simulink model "pfc"  (R2018b)
settings: Solver=VariableStepAuto  StartTime=0.0  StopTime=1  RelTol=1e-3
InitFcn:
  | % Time %
  | fpwm = 18e3
  | fs = fpwm
  | Ts = 1/fs
  | 
  | %pfc Current Loop - plant is only inductance%
  | Vin_ac = 264
  | Cin = 2.2e-6
  | Vin_peak = 1.414 * Vin_ac
  | Vin_dc = Vin_peak
  | Rshunt = 20e-3
  | L = 3e-3
  | R = 0.123
  | BW_Ipfc = 1400
  | Vmax = Vin_dc  % max applied Vplant %
  | Gain_Ipfc = (Vmax / 1)  % (Vplant / Ipfc_dutycycle) %
  | Kp_Ipfc = (2*pi*BW_Ipfc * L) / Gain_Ipfc
  | Ki_Ipfc = (2*pi*BW_Ipfc * R) / Gain_Ipfc
  | 
  | % pfc Voltage Loop %
  | Cdc = 1080e-6
  | Vc_init = 0.8*Vin_peak  % initial capacitor voltage %
  | Rload = 80
  | BW_Vpfc = 10
  | Gain_Vpfc = 1  % V_loop_PI_out to Iref_pfc %
  | Kp_Vpfc = (2*pi*BW_Vpfc * Cdc) / Gain_Vpfc
  | Ki_Vpfc = (2*pi*BW_Vpfc / Rload) / Gain_Vpfc
  | Gain_ffV = 0.25   % feed forward gain %
libraries: powerlib x17, dspstat3 x3, simulink x2, powerlib_meascontrol x1
settings Model: Creator=GURU SEKHAR  LastModifiedBy=GURU SEKHAR

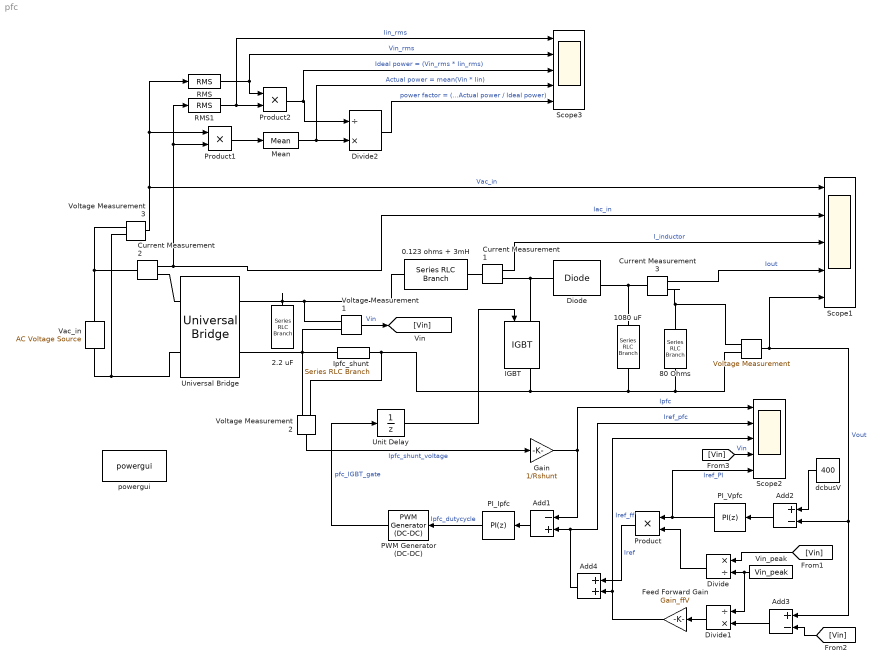
== system pfc ==
  "                       " : powerlib/Measurements/Voltage Measurement  PhasorSimulation=off  OutputType=Complex  PSBequivalent=0
  0.123 ohms + 3mH : powerlib/Elements/Series RLC Branch  LConnTagsString=__new0  RConnTagsString=__new0  BranchType=RL  Resistance=R  Inductance=L  SetiL0=off  InitialCurrent=0  Capacitance=1e-6  Setx0=off  InitialVoltage=0  Measurements=None
  1080 uF : powerlib/Elements/Series RLC Branch  LConnTagsString=__new0  RConnTagsString=__new0  BranchType=C  Resistance=1  Inductance=1e-3  SetiL0=off  InitialCurrent=0  Capacitance=Cdc  Setx0=on  InitialVoltage=Vc_init  Measurements=None
  2.2 uF : powerlib/Elements/Series RLC Branch  LConnTagsString=__new0  RConnTagsString=__new0  BranchType=C  Resistance=1  Inductance=1e-3  SetiL0=off  InitialCurrent=0  Capacitance=Cin  Setx0=off  InitialVoltage=Vc_init  Measurements=None
  "80 Ohms " : powerlib/Elements/Series RLC Branch  LConnTagsString=__new0  RConnTagsString=__new0  BranchType=R  Resistance=80  Inductance=1e-3  SetiL0=off  InitialCurrent=0  Capacitance=1e-6  Setx0=off  InitialVoltage=0  Measurements=None
  Add1 : Sum  Inputs=-+
  Add2 : Sum  Inputs=+-
  Add3 : Sum  Inputs=+-
  Add4 : Sum
  Current Measurement1 : powerlib/Measurements/Current Measurement  PhasorSimulation=off  OutputType=Complex  PSBequivalent=0
  Current Measurement2 : powerlib/Measurements/Current Measurement  PhasorSimulation=off  OutputType=Complex  PSBequivalent=0
  Current Measurement3 : powerlib/Measurements/Current Measurement  PhasorSimulation=off  OutputType=Complex  PSBequivalent=0
  Diode : powerlib/Power Electronics/Diode  Ron=0.001  Lon=0  Vf=0.8  IC=0  UseSnubber=off  Rs=500  Cs=250e-9  Measurements=on
  Divide : Product  Inputs=*/
  Divide1 : Product  Inputs=/*
  Divide2 : Product  Inputs=/*
  Feed Forward Gain : Gain  Gain=Gain_ffV
  Gain : Gain  Gain=1/Rshunt
  IGBT : powerlib/Power Electronics/IGBT  Ron=0.001  Lon=0  Vf=1  Tf=1e-6  Tt=2e-6  IC=0  Rs=1e5  Cs=inf  Measurements=on
  Ipfc_shunt : powerlib/Elements/Series RLC Branch  LConnTagsString=__new0  RConnTagsString=__new0  BranchType=R  Resistance=Rshunt  Inductance=1e-3  SetiL0=off  InitialCurrent=0  Capacitance=1e-6  Setx0=off  InitialVoltage=0  Measurements=None
  Mean : dspstat3/Mean  run=on  reset_popup=None  directionMode=Each column  dimension=1  roiEnable=off  roiType=Rectangles  roiPortion=Entire ROI  roiOutput=Individual statistics for each ROI  roiFlag=off  roundingMode=Floor  overflowMode=off  outputDataTypeStr=Inherit: Same as accumulator  outputMin=[]  outputMax=[]  outputLastDataTypeStr=Inherit: Same as accumulator
  PI_Ipfc : simulink/Continuous/PID Controller  Controller=PI  Form=Parallel  TimeDomain=Discrete-time  SampleTime=-1  IntegratorMethod=Forward Euler  FilterMethod=Forward Euler  ControllerParametersSource=internal  P=Kp_Ipfc  I=Ki_Ipfc  D=0  UseFilter=on  N=100  TunerSelectOption=Transfer Function Based (PID Tuner App)  InitialConditionSource=internal  InitialConditionForIntegrator=0  InitialConditionForFilter=0  DifferentiatorICPrevScaledInput=0  ExternalReset=none  TrackingMode=off  Kt=1  LimitOutput=on  UpperSaturationLimit=1  LowerSaturationLimit=0  LinearizeAsGain=on  AntiWindupMode=clamping  Kb=1  POutMin=[]  POutMax=[]  IOutMin=[]  IOutMax=[]  DOutMin=[]  DOutMax=[]  NOutMin=[]  NOutMax=[]  SumOutMin=[]  SumOutMax=[]  SaturationOutMin=[]  SaturationOutMax=[]  PParamMin=[]  PParamMax=[]  IParamMin=[]  IParamMax=[]  DParamMin=[]  DParamMax=[]  NParamMin=[]  NParamMax=[]  KbParamMin=[]  KbParamMax=[]  KtParamMin=[]  KtParamMax=[]  KbOutMin=[]  KbOutMax=[]  KtOutMin=[]  KtOutMax=[]  IntegratorOutMin=[]  IntegratorOutMax=[]  FilterOutMin=[]  FilterOutMax=[]  SumI1OutMin=[]  SumI1OutMax=[]  SumI2OutMin=[]  SumI2OutMax=[]  SumI3OutMin=[]  SumI3OutMax=[]  SumI4OutMin=[]  SumI4OutMax=[]  SumDOutMin=[]  SumDOutMax=[]  DifferentiatorOutMin=[]  DifferentiatorOutMax=[]  FilterDiffOutCoefMin=[]  FilterDiffOutCoefMax=[]  ReciprocalOutMin=[]  ReciprocalOutMax=[]  SumDenOutMin=[]  SumDenOutMax=[]  SumNumOutMin=[]  SumNumOutMax=[]  DivideOutMin=[]  DivideOutMax=[]  IntegratorContinuousStateAttributes=''  IntegratorStateMustResolveToSignalObject=off  IntegratorRTWStateStorageClass=Auto  FilterContinuousStateAttributes=''  FilterStateMustResolveToSignalObject=off  FilterRTWStateStorageClass=Auto  ParallelPVariant=InternalParameters  IdealPVariant=Disabled  IVariant=InternalParameters  DVariant=Disabled  IntegratorVariant=Discrete  SatVariant=Enabled  AWVariant=DiscClampingParallel  PCopyVariant=Disabled  TRVariant=Disabled  FdbkBlocksVariant=Forward  IdealPFdbkVariant=Disabled  SatFdbkVariant=Disabled  DerivativeFilterVariant=Disabled  NVariant=Disabled  NCopyVariant=Disabled_SignalSpec  FilterICVariant=Disabled  IntegratorICVariant=InternalICs  ExternalResetVariant=Disabled  TRSumVariant=Passthrough  SumFdbkVariant=Disabled  SumVariant=Sum_PI
  PI_Vpfc : simulink/Continuous/PID Controller  Controller=PI  Form=Parallel  TimeDomain=Discrete-time  SampleTime=-1  IntegratorMethod=Forward Euler  FilterMethod=Forward Euler  ControllerParametersSource=internal  P=Kp_Vpfc  I=Ki_Vpfc  D=0  UseFilter=on  N=100  TunerSelectOption=Transfer Function Based (PID Tuner App)  InitialConditionSource=internal  InitialConditionForIntegrator=0  InitialConditionForFilter=0  DifferentiatorICPrevScaledInput=0  ExternalReset=none  TrackingMode=off  Kt=1  LimitOutput=on  UpperSaturationLimit=50  LowerSaturationLimit=0  LinearizeAsGain=on  AntiWindupMode=clamping  Kb=1  POutMin=[]  POutMax=[]  IOutMin=[]  IOutMax=[]  DOutMin=[]  DOutMax=[]  NOutMin=[]  NOutMax=[]  SumOutMin=[]  SumOutMax=[]  SaturationOutMin=[]  SaturationOutMax=[]  PParamMin=[]  PParamMax=[]  IParamMin=[]  IParamMax=[]  DParamMin=[]  DParamMax=[]  NParamMin=[]  NParamMax=[]  KbParamMin=[]  KbParamMax=[]  KtParamMin=[]  KtParamMax=[]  KbOutMin=[]  KbOutMax=[]  KtOutMin=[]  KtOutMax=[]  IntegratorOutMin=[]  IntegratorOutMax=[]  FilterOutMin=[]  FilterOutMax=[]  SumI1OutMin=[]  SumI1OutMax=[]  SumI2OutMin=[]  SumI2OutMax=[]  SumI3OutMin=[]  SumI3OutMax=[]  SumI4OutMin=[]  SumI4OutMax=[]  SumDOutMin=[]  SumDOutMax=[]  DifferentiatorOutMin=[]  DifferentiatorOutMax=[]  FilterDiffOutCoefMin=[]  FilterDiffOutCoefMax=[]  ReciprocalOutMin=[]  ReciprocalOutMax=[]  SumDenOutMin=[]  SumDenOutMax=[]  SumNumOutMin=[]  SumNumOutMax=[]  DivideOutMin=[]  DivideOutMax=[]  IntegratorContinuousStateAttributes=''  IntegratorStateMustResolveToSignalObject=off  IntegratorRTWStateStorageClass=Auto  FilterContinuousStateAttributes=''  FilterStateMustResolveToSignalObject=off  FilterRTWStateStorageClass=Auto  ParallelPVariant=InternalParameters  IdealPVariant=Disabled  IVariant=InternalParameters  DVariant=Disabled  IntegratorVariant=Discrete  SatVariant=Enabled  AWVariant=DiscClampingParallel  PCopyVariant=Disabled  TRVariant=Disabled  FdbkBlocksVariant=Forward  IdealPFdbkVariant=Disabled  SatFdbkVariant=Disabled  DerivativeFilterVariant=Disabled  NVariant=Disabled  NCopyVariant=Disabled_SignalSpec  FilterICVariant=Disabled  IntegratorICVariant=InternalICs  ExternalResetVariant=Disabled  TRSumVariant=Passthrough  SumFdbkVariant=Disabled  SumVariant=Sum_PI
  PWM Generator (DC-DC) : powerlib_meascontrol/Pulse & Signal Generators/PWM Generator (DC-DC)  Fsw=fpwm  Ts=Ts
  Product : Product
  Product1 : Product
  Product2 : Product
  RMS : dspstat3/RMS  run=on  directionMode=Each column  dimension=1  reset_popup=None
  RMS1 : dspstat3/RMS  run=on  directionMode=Each column  dimension=1  reset_popup=None
  Scope1 : Scope  NumInputPorts=5
  Scope2 : Scope  NumInputPorts=5
  Scope3 : Scope  NumInputPorts=5
  Unit Delay : UnitDelay  SampleTime=-1
  Universal Bridge : powerlib/Power Electronics/Universal Bridge  Arms=2  SnubberResistance=1e5  SnubberCapacitance=inf  Device=Diodes  Ron=1e-3  Lon=0  ForwardVoltages="[  0  0  ]"  ForwardVoltage=0  GTOparameters=[ 10e-6 , 20e-6 ]  IGBTparameters=[ 1e-6 , 2e-6 ]  Measurements=None  Measurements_2=None  converterType=Rectifier
  Vac_in : powerlib/Electrical Sources/AC Voltage Source  Amplitude=Vin_ac * 1.414  Phase=0  Frequency=50  SampleTime=-1  Measurements=None  BusType=swing  Pref=10e3  Qref=0  Qmin=-inf  Qmax=+inf
  Vin_peak : Constant  Value=Vin_peak  SampleTime=-1
  Voltage Measurement1 : powerlib/Measurements/Voltage Measurement  PhasorSimulation=off  OutputType=Complex  PSBequivalent=0
  Voltage Measurement2 : powerlib/Measurements/Voltage Measurement  PhasorSimulation=off  OutputType=Complex  PSBequivalent=0
  Voltage Measurement3 : powerlib/Measurements/Voltage Measurement  PhasorSimulation=off  OutputType=Complex  PSBequivalent=0
  dcbusV : Constant  Value=400
  powergui : powerlib/powergui  Priority=1  SimulationMode=Discrete  SampleTime=Ts  frequency=60  Iterations=50  frequencyindice=50  Pbase=100e6  ErrMax=1e-4  UnitsV=kV  UnitsW=MW  buscounter=0  FunctionMessages=off  echomessages=off  EnableUseOfTLC=off  CurrentSourceSwitches=off  DisableSnubberDevices=off  DisableRonSwitches=off  DisableVfSwitches=off  DisplayEquations=off  SolverType=Tustin/Backward Euler (TBE)  Interpol=off  ExternalGateDelay=off  methode=off  Ts=100  x0status=blocks  SPID=on  SwTol=0  HookPort=off  RestoreLinks=warning  ResistiveCurrentMeasurement=off  Frange=[0:2:500]  Ylog=off  Xlog=on  ShowGrid=off  save=off  variable=ZData  structure=0  ZoomFFT=off  StartTime=0.0  cycles=1  DisplayStyle=1  fundamental=60  FreqAxis=off  MaxFrequency=1000  frequencyindicesteady=1  RmsSteady=1  display=off
  wires:
  RMS1/1 -> Product2/2, Scope3/1  "Iin_rms"
  Mean/1 -> Scope3/4, Divide2/2  "Actual power = mean(Vin * Iin)"
  Divide2/1 -> Scope3/5  "power factor = (Actual power / Ideal power)"
  Product/1 -> Add4/1  "Iref"
  Add2/1 -> PI_Vpfc/1
  Product2/1 -> Scope3/3, Divide2/1  "Ideal power = (Vin_rms * Iin_rms)"
  Voltage Measurement3/1 -> Product1/1, RMS/1, Scope1/1  "Vac_in"
  dcbusV/1 -> Add2/1
  Add4/1 -> Scope2/2, Add1/2  "Iref_pfc"
  Current Measurement2/1 -> RMS1/1, Product1/2, Scope1/2  "Iac_in"
  PI_Ipfc/1 -> PWM Generator (DC-DC)/1  "Ipfc_dutycycle"
  Product1/1 -> Mean/1
  Feed Forward Gain/1 -> Scope2/3, Add4/2  "Iref_ff"
  [Vin] -> Divide/1
  PI_Vpfc/1 -> Scope2/5, Product/1  "Iref_PI"
  Voltage Measurement1/1 -> [Vin]  "Vin"
  Unit Delay/1 -> IGBT/1
  Vin_peak/1 -> Divide1/1, Divide/2
  Current Measurement1/1 -> Scope1/3  "I_inductor"
  Add3/1 -> Divide1/2
  [Vin] -> Add3/2
  PWM Generator (DC-DC)/1 -> Unit Delay/1  "pfc_IGBT_gate"
  Current Measurement3/1 -> Scope1/4  "Iout"
  RMS/1 -> Product2/1, Scope3/2  "Vin_rms"
  [Vin] -> Scope2/4  "Vin"
  Add1/1 -> PI_Ipfc/1
  Voltage Measurement2/1 -> Gain/1  "Ipfc_shunt_voltage"
  Divide1/1 -> Feed Forward Gain/1
  "                       "/1 -> Scope1/5, Add3/1, Add2/2  "Vout"
  Gain/1 -> Scope2/1, Add1/1  "Ipfc"
  Divide/1 -> Product/2
  connections:
  Universal Bridge/LConn2 -- Vac_in/LConn1 -- Voltage Measurement3/LConn2
  Voltage Measurement3/LConn1 -- Current Measurement2/LConn1 -- Vac_in/RConn1
  Diode/RConn1 -- Current Measurement3/LConn1 -- 1080 uF/LConn1
  Voltage Measurement1/LConn2 -- Universal Bridge/RConn2 -- Ipfc_shunt/LConn1 -- Voltage Measurement2/LConn2
  "80 Ohms "/LConn1 -- "                       "/LConn1 -- Current Measurement3/RConn1
  1080 uF/RConn1 -- Voltage Measurement2/LConn1 -- Ipfc_shunt/RConn1 -- IGBT/RConn1 -- "80 Ohms "/RConn1 -- "                       "/LConn2
  Diode/LConn1 -- IGBT/LConn1 -- Current Measurement1/RConn1
  2.2 uF/LConn1 -- Voltage Measurement1/LConn1 -- 0.123 ohms + 3mH/LConn1 -- Universal Bridge/RConn1
  Current Measurement1/LConn1 -- 0.123 ohms + 3mH/RConn1
  Current Measurement2/RConn1 -- Universal Bridge/LConn1
